simulink model "test_trajectory"  (R2015a)
settings: Solver=ode45  StartTime=0.0  StopTime=30.0  RelTol=1e-3
undefined symbols (not defined in the file): L1, v
settings Model: Creator=Sara  LastModifiedBy=Sara

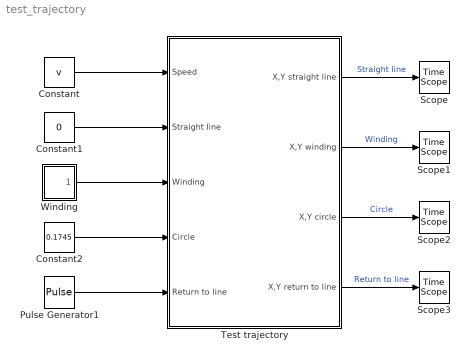
== system test_trajectory ==
  Constant : Constant  Value=v
  Constant1 : Constant  Value=0
  Constant2 : Constant  Value=0.1745
  Pulse Generator1 : DiscretePulseGenerator  PulseType=Time based  Amplitude=0.7853  Period=10  PulseWidth=50  PhaseDelay=5
  Scope{,1..3} (4 alike) : TimeScope
  Test trajectory : Subsystem
  Winding : Subsystem
  wires:
  Constant/1 -> Test trajectory/1(Speed)
  Test trajectory/1(X,Y straight line) -> Scope/1  "Straight line"
  Constant1/1 -> Test trajectory/2(Straight line)
  Constant2/1 -> Test trajectory/4(Circle)
  Pulse Generator1/1 -> Test trajectory/5(Return to line)
  Test trajectory/4(X,Y return to line) -> Scope3/1  "Return to line"
  Test trajectory/3(X,Y circle) -> Scope2/1  "Circle"
  Test trajectory/2(X,Y winding) -> Scope1/1  "Winding"
  Winding/1(Out1) -> Test trajectory/3(Winding)

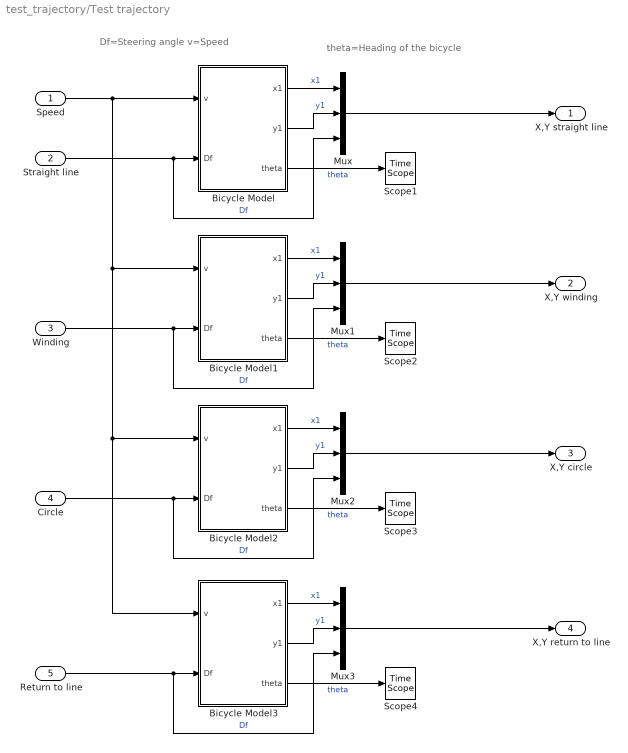
== system test_trajectory/Test trajectory ==
  note: Df=Steering angle
      | v=Speed
  note: theta=Heading of the bicycle
  Speed : Inport
  Straight line : Inport  Port=2
  Winding : Inport  Port=3
  Circle : Inport  Port=4
  Return to line : Inport  Port=5
  Bicycle Model : Subsystem
  Bicycle Model1 : Subsystem
  Bicycle Model2 : Subsystem
  Bicycle Model3 : Subsystem
  Mux{,1..3} (4 alike) : Mux  Inputs=3
  Scope{1..4} (4 alike) : TimeScope
  X,Y straight line : Outport
  X,Y winding : Outport  Port=2
  X,Y circle : Outport  Port=3
  X,Y return to line : Outport  Port=4
  wires:
  Bicycle Model/1(x1) -> Mux/1  "x1"
  Bicycle Model/3(theta) -> Scope1/1  "theta"
  Bicycle Model/2(y1) -> Mux/2  "y1"
  Mux/1 -> X,Y straight line/1
  Straight line/1 -> Mux/3, Bicycle Model/2(Df)  "Df"
  Bicycle Model1/1(x1) -> Mux1/1  "x1"
  Bicycle Model1/3(theta) -> Scope2/1  "theta"
  Bicycle Model1/2(y1) -> Mux1/2  "y1"
  Winding/1 -> Bicycle Model1/2(Df), Mux1/3  "Df"
  Mux1/1 -> X,Y winding/1
  Bicycle Model2/1(x1) -> Mux2/1  "x1"
  Bicycle Model2/3(theta) -> Scope3/1  "theta"
  Bicycle Model2/2(y1) -> Mux2/2  "y1"
  Circle/1 -> Mux2/3, Bicycle Model2/2(Df)  "Df"
  Mux2/1 -> X,Y circle/1
  Bicycle Model3/1(x1) -> Mux3/1  "x1"
  Speed/1 -> Bicycle Model3/1(v), Bicycle Model2/1(v), Bicycle Model1/1(v), Bicycle Model/1(v)
  Bicycle Model3/3(theta) -> Scope4/1  "theta"
  Bicycle Model3/2(y1) -> Mux3/2  "y1"
  Return to line/1 -> Bicycle Model3/2(Df), Mux3/3  "Df"
  Mux3/1 -> X,Y return to line/1

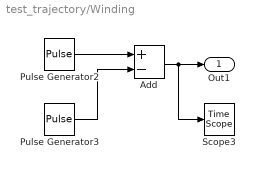
== system test_trajectory/Winding ==
  Add : Sum  Inputs=+-
  Pulse Generator2 : DiscretePulseGenerator  PulseType=Time based  Amplitude=0.2617  Period=10  PulseWidth=50
  Pulse Generator3 : DiscretePulseGenerator  PulseType=Time based  Amplitude=0.2617  Period=10  PulseWidth=50  PhaseDelay=2.5
  Scope3 : TimeScope
  Out1 : Outport
  wires:
  Pulse Generator2/1 -> Add/1
  Pulse Generator3/1 -> Add/2
  Add/1 -> Scope3/1, Out1/1

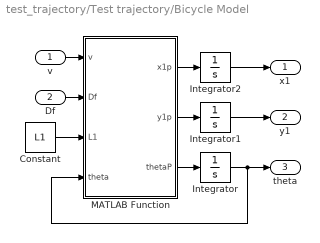
== system test_trajectory/Test trajectory/Bicycle Model ==
  v : Inport
  Df : Inport  Port=2
  Constant : Constant  Value=L1
  Integrator : Integrator
  Integrator1 : Integrator
  Integrator2 : Integrator
  MATLAB Function : MATLAB Function  TreatAsAtomicUnit=on
  x1 : Outport
  y1 : Outport  Port=2
  theta : Outport  Port=3
  wires:
  MATLAB Function/1(x1p) -> Integrator2/1
  MATLAB Function/3(thetaP) -> Integrator/1
  Integrator1/1 -> y1/1
  v/1 -> MATLAB Function/1(v)
  Integrator2/1 -> x1/1
  Df/1 -> MATLAB Function/2(Df)
  Integrator/1 -> MATLAB Function/4(theta), theta/1
  MATLAB Function/2(y1p) -> Integrator1/1
  Constant/1 -> MATLAB Function/3(L1)

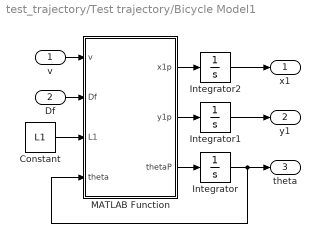
== system test_trajectory/Test trajectory/Bicycle Model1 ==
  v : Inport
  Df : Inport  Port=2
  Constant : Constant  Value=L1
  Integrator : Integrator
  Integrator1 : Integrator
  Integrator2 : Integrator
  MATLAB Function : MATLAB Function  TreatAsAtomicUnit=on
  x1 : Outport
  y1 : Outport  Port=2
  theta : Outport  Port=3
  wires:
  Constant/1 -> MATLAB Function/3(L1)
  MATLAB Function/2(y1p) -> Integrator1/1
  Integrator/1 -> theta/1, MATLAB Function/4(theta)
  Df/1 -> MATLAB Function/2(Df)
  Integrator2/1 -> x1/1
  v/1 -> MATLAB Function/1(v)
  Integrator1/1 -> y1/1
  MATLAB Function/3(thetaP) -> Integrator/1
  MATLAB Function/1(x1p) -> Integrator2/1

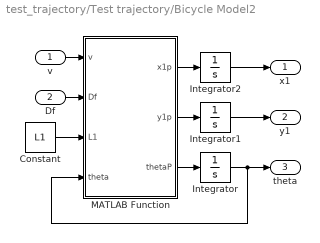
== system test_trajectory/Test trajectory/Bicycle Model2 ==
  v : Inport
  Df : Inport  Port=2
  Constant : Constant  Value=L1
  Integrator : Integrator
  Integrator1 : Integrator
  Integrator2 : Integrator
  MATLAB Function : MATLAB Function  TreatAsAtomicUnit=on
  x1 : Outport
  y1 : Outport  Port=2
  theta : Outport  Port=3
  wires:
  MATLAB Function/1(x1p) -> Integrator2/1
  MATLAB Function/3(thetaP) -> Integrator/1
  Integrator1/1 -> y1/1
  v/1 -> MATLAB Function/1(v)
  Integrator2/1 -> x1/1
  Df/1 -> MATLAB Function/2(Df)
  Integrator/1 -> MATLAB Function/4(theta), theta/1
  MATLAB Function/2(y1p) -> Integrator1/1
  Constant/1 -> MATLAB Function/3(L1)

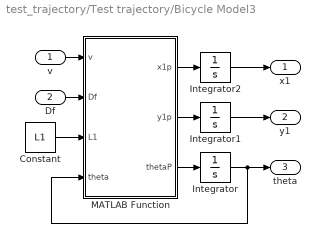
== system test_trajectory/Test trajectory/Bicycle Model3 ==
  v : Inport
  Df : Inport  Port=2
  Constant : Constant  Value=L1
  Integrator : Integrator
  Integrator1 : Integrator
  Integrator2 : Integrator
  MATLAB Function : MATLAB Function  TreatAsAtomicUnit=on
  x1 : Outport
  y1 : Outport  Port=2
  theta : Outport  Port=3
  wires:
  Constant/1 -> MATLAB Function/3(L1)
  MATLAB Function/2(y1p) -> Integrator1/1
  Integrator/1 -> theta/1, MATLAB Function/4(theta)
  Df/1 -> MATLAB Function/2(Df)
  Integrator2/1 -> x1/1
  v/1 -> MATLAB Function/1(v)
  Integrator1/1 -> y1/1
  MATLAB Function/3(thetaP) -> Integrator/1
  MATLAB Function/1(x1p) -> Integrator2/1

== matlab function test_trajectory/Test trajectory/Bicycle Model1/MATLAB Function ==
  data: x1p output; y1p output; v input; thetaP output; Df input; L1 input; theta input
function [x1p,y1p,thetaP] = fcn(v,Df,L1,theta)
%Rotation rate equation
thetaP=(v*sin(Df))/L1;

x1p=v*cos(theta+Df);
y1p=v*sin(theta+Df);

== matlab function test_trajectory/Test trajectory/Bicycle Model/MATLAB Function ==
  data: x1p output; y1p output; v input; thetaP output; Df input; L1 input; theta input
function [x1p,y1p,thetaP] = fcn(v,Df,L1,theta)
%Rotation rate equation
thetaP=(v*sin(Df))/L1;

x1p=v*cos(theta+Df);
y1p=v*sin(theta+Df);

== matlab function test_trajectory/Test trajectory/Bicycle Model2/MATLAB Function ==
  data: x1p output; y1p output; v input; thetaP output; Df input; L1 input; theta input
function [x1p,y1p,thetaP] = fcn(v,Df,L1,theta)
%Rotation rate equation
thetaP=(v*sin(Df))/L1;

x1p=v*cos(theta+Df);
y1p=v*sin(theta+Df);

== matlab function test_trajectory/Test trajectory/Bicycle Model3/MATLAB Function ==
  data: x1p output; y1p output; v input; thetaP output; Df input; L1 input; theta input
function [x1p,y1p,thetaP] = fcn(v,Df,L1,theta)
%Rotation rate equation
thetaP=(v*sin(Df))/L1;

x1p=v*cos(theta+Df);
y1p=v*sin(theta+Df);
